simulink model "QaternionModel"  (R2012b)
settings: Solver=ode45  StartTime=0.0  StopTime=20  RelTol=1e-3
libraries: aerolibutil x6, aerolibtransform2 x6, vrlib x2, dspmtrx3 x1
settings Model: Creator=Mirag_000  LastModifiedBy=Mirag_000
settings DataIOCC: SignalLoggingSaveFormat=ModelDataLogs
settings OptimizationCC: ExpressionDepthLimit=128
settings DebuggingCC: MultiTaskDSMMsg=warning  MultiTaskCondExecSysMsg=none  StrictBusMsg=None
settings RTWCC: IncludeERTFirstTime=on
settings CodeAppCC: CustomSymbolStrType=$N$R$M_T  InternalIdentifier=Shortened

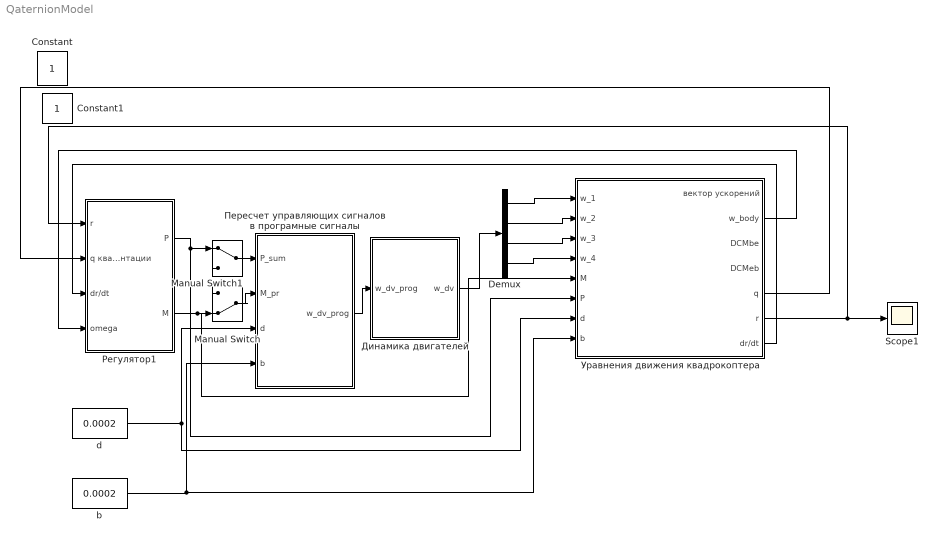
== system QaternionModel ==
  Demux : Demux
  Manual Switch : ManualSwitch  CurrentSetting=0
  Manual Switch1 : ManualSwitch
  Scope1 : Scope
  b : Constant  Value=0.0002
  d : Constant  Value=0.0002
  Динамика двигателей : Subsystem
  Пересчет управляющих сигналов в програмные сигналы : Subsystem
  Регулятор1 : Subsystem
  Уравнения движения квадрокоптера : Subsystem
  Constant : Constant  IOType=siggen  VectorParams1D=off  SampleTime=1
  Constant1 : Constant  IOType=siggen
  wires:
  Demux/1 -> Уравнения движения квадрокоптера/1(w_1)
  Demux/2 -> Уравнения движения квадрокоптера/2(w_2)
  Demux/3 -> Уравнения движения квадрокоптера/3(w_3)
  Demux/4 -> Уравнения движения квадрокоптера/4(w_4)
  Уравнения движения квадрокоптера/6(r) -> Регулятор1/1(r), Scope1/1
  Пересчет управляющих сигналов в програмные сигналы/1(w_dv_prog) -> Динамика двигателей/1(w_dv_prog)
  Уравнения движения квадрокоптера/5(q) -> Регулятор1/2(q кватернион текущей ориентации)
  Уравнения движения квадрокоптера/7(dr/dt) -> Регулятор1/3(dr/dt)
  Уравнения движения квадрокоптера/2(w_body) -> Регулятор1/4(omega)
  Регулятор1/1(P) -> Manual Switch1/1, Уравнения движения квадрокоптера/6(P)
  Регулятор1/2(M) -> Уравнения движения квадрокоптера/5(M), Manual Switch/2
  Динамика двигателей/1(w_dv) -> Demux/1
  Manual Switch1/1 -> Пересчет управляющих сигналов в програмные сигналы/1(P_sum)
  Manual Switch/1 -> Пересчет управляющих сигналов в програмные сигналы/2(M_pr)
  d/1 -> Пересчет управляющих сигналов в програмные сигналы/3(d), Уравнения движения квадрокоптера/7(d)
  b/1 -> Уравнения движения квадрокоптера/8(b), Пересчет управляющих сигналов в програмные сигналы/4(b)

== system QaternionModel/Динамика двигателей ==
  w_dv_prog : Inport
  Demux1 : Demux
  Manual Switch : ManualSwitch
  Scope : Scope
      settings: SaveName=ScopeData32
  Transfer Fcn{4..7} (4 alike) : TransferFcn  Denominator=[0.003 1]
  Vector Concatenate1 : Concatenate  NumInputs=4
  w_dv : Outport
  wires:
  Manual Switch/1 -> w_dv/1
  w_dv_prog/1 -> Demux1/1
  Transfer Fcn5/1 -> Vector Concatenate1/2
  Transfer Fcn6/1 -> Vector Concatenate1/3
  Transfer Fcn7/1 -> Vector Concatenate1/4
  Demux1/1 -> Transfer Fcn4/1
  Transfer Fcn4/1 -> Vector Concatenate1/1
  Demux1/2 -> Transfer Fcn5/1
  Demux1/3 -> Transfer Fcn6/1
  Demux1/4 -> Transfer Fcn7/1
  Vector Concatenate1/1 -> Scope/1, Manual Switch/1

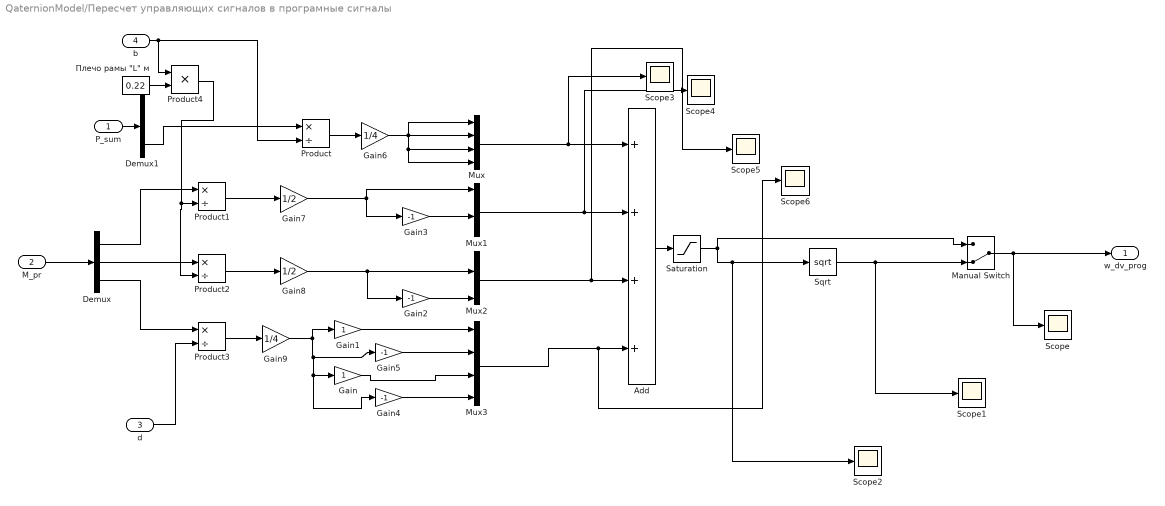
== system QaternionModel/Пересчет управляющих сигналов в програмные сигналы ==
  P_sum : Inport
  M_pr : Inport  Port=2
  d : Inport  Port=3
  b : Inport  Port=4
  Add : Sum  Inputs=++++
  Demux : Demux  Outputs=3
  Demux1 : Demux  Outputs=3
  Gain : Gain
  Gain1 : Gain
  Gain{2..5} (4 alike) : Gain  Gain=-1
  Gain6 : Gain  Gain=1/4
  Gain7 : Gain  Gain=1/2
  Gain8 : Gain  Gain=1/2
  Gain9 : Gain  Gain=1/4
  Manual Switch : ManualSwitch  CurrentSetting=0
  Mux{,1..3} (4 alike) : Mux
  Product{,1..3} (4 alike) : Product  Inputs=*/
  Product4 : Product
  Saturation : Saturate  UpperLimit=50000  LowerLimit=0.001
  Scope{,1..6} (7 alike) : Scope
      Scope settings: YMin=1.6575  YMax=1.6775  SaveName=ScopeData20
      Scope1 settings: YMin=60  YMax=180  SaveName=ScopeData34
      Scope2 settings: YMin=0.07  YMax=0.1025  SaveName=ScopeData44
      Scope3 settings: YMin=60  YMax=180  SaveName=ScopeData23
      Scope4 settings: YMin=60  YMax=180  SaveName=ScopeData24
      Scope5 settings: YMin=60  YMax=180  SaveName=ScopeData27
      Scope6 settings: YMin=60  YMax=180  SaveName=ScopeData28
  Sqrt : Sqrt  SaturateOnIntegerOverflow=on
  "Плечо рамы \"L\" м" : Constant  Value=0.22
  w_dv_prog : Outport
  wires:
  Gain/1 -> Mux3/3
  Gain1/1 -> Mux3/1
  Product3/1 -> Gain9/1
  Product2/1 -> Gain8/1
  Gain2/1 -> Mux2/4
  Gain3/1 -> Mux1/3
  Product1/1 -> Gain7/1
  Product/1 -> Gain6/1
  Mux2/1 -> Scope5/1, Add/3
  Mux1/1 -> Scope4/1, Add/2
  Mux/1 -> Scope3/1, Add/1
  Mux3/1 -> Scope6/1, Add/4
  Gain5/1 -> Mux3/2
  Gain4/1 -> Mux3/4
  Sqrt/1 -> Scope1/1, Manual Switch/2
  Demux/1 -> Product1/1
  Demux/2 -> Product2/1
  d/1 -> Product3/2
  "Плечо рамы \"L\" м"/1 -> Product4/2
  b/1 -> Product/2, Product4/1
  Product4/1 -> Product2/2, Product1/2
  Gain6/1 -> Mux/4, Mux/3, Mux/1, Mux/2
  Gain7/1 -> Gain3/1, Mux1/1
  Gain8/1 -> Gain2/1, Mux2/2
  Gain9/1 -> Gain1/1, Gain4/1, Gain/1, Gain5/1
  Demux/3 -> Product3/1
  M_pr/1 -> Demux/1
  P_sum/1 -> Demux1/1
  Demux1/3 -> Product/1
  Manual Switch/1 -> w_dv_prog/1, Scope/1
  Add/1 -> Saturation/1
  Saturation/1 -> Manual Switch/1, Scope2/1, Sqrt/1

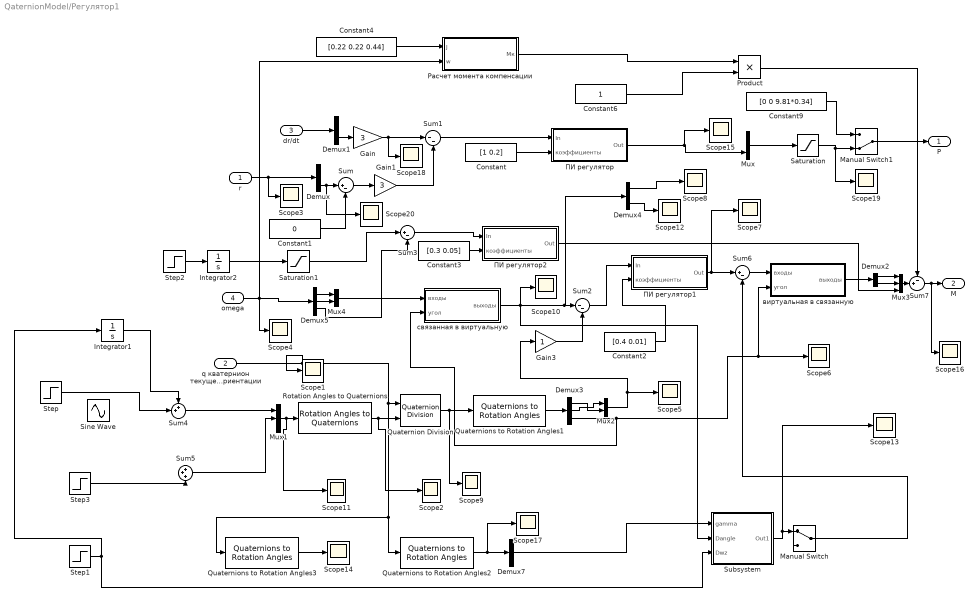
== system QaternionModel/Регулятор1 ==
  r : Inport
  q кватернион текущей ориентации : Inport  Port=2
  dr/dt : Inport  Port=3
  omega : Inport  Port=4
  Constant : Constant  Value=[1 0.2]
  Constant1 : Constant  Value=0
  Constant2 : Constant  Value=[0.4 0.01]
  Constant3 : Constant  Value=[0.3 0.05]
  Constant4 : Constant  Value=[0.22 0.22 0.44]
  Constant6 : Constant
  Constant9 : Constant  Value=[0 0 9.81*0.34]
  Demux{,1,3,5,7} (5 alike) : Demux  Outputs=3
  Demux2 : Demux  Outputs=2
  Demux4 : Demux  Outputs=2
  Gain : Gain  Gain=3
  Gain1 : Gain  Gain=3
  Gain3 : Gain
  Integrator1 : Integrator
  Integrator2 : Integrator
  Manual Switch : ManualSwitch
  Manual Switch1 : ManualSwitch  CurrentSetting=0
  Mux : Mux  Inputs=3
  Mux1 : Mux  Inputs=3
  Mux2 : Mux  Inputs=2
  Mux3 : Mux  Inputs=3
  Mux4 : Mux  Inputs=2
  Product : Product  RndMeth=Zero
  Quaternion Division : aerolibutil/Quaternion Division
  Quaternions to Rotation Angles1 : aerolibtransform2/Quaternions to Rotation Angles  rotationOrder=YXZ
  Quaternions to Rotation Angles2 : aerolibtransform2/Quaternions to Rotation Angles  rotationOrder=ZYZ
  Quaternions to Rotation Angles3 : aerolibtransform2/Quaternions to Rotation Angles  rotationOrder=ZYZ
  Rotation Angles to Quaternions : aerolibtransform2/Rotation Angles to Quaternions  rotationOrder=ZYX
  Saturation : Saturate  UpperLimit=100  LowerLimit=0
  Saturation1 : Saturate  UpperLimit=3  LowerLimit=0
  Scope{1..20} (20 alike) : Scope
      Scope1 settings: SaveName=ScopeData2
      Scope10 settings: YMin=-0.008  YMax=0.008  SaveName=ScopeData12
      Scope11 settings: YMin=-1  YMax=0.1  SaveName=ScopeData14
      Scope12 settings: YMin=-2.75  YMax=1.5  SaveName=ScopeData17
      Scope13 settings: YMin=-2.75  YMax=1.5  SaveName=ScopeData21
      Scope14 settings: TimeRange=18.29822608393934  YMin=0.993671875  YMax=1.008984375  SaveName=ScopeData22
      Scope15 settings: YMin=-2.75  YMax=1.5  SaveName=ScopeData10
      Scope16 settings: YMin=-2.75  YMax=1.5  SaveName=ScopeData29
      Scope17 settings: TimeRange=18.29822608393934  YMin=0.993671875  YMax=1.008984375  SaveName=ScopeData25
      Scope18 settings: SaveName=ScopeData30
      Scope19 settings: TimeRange=20  YMin=-2.75  YMax=1.5  SaveName=ScopeData31
      Scope2 settings: YMin=-1  YMax=0.1  SaveName=ScopeData3
      Scope20 settings: SaveName=ScopeData33
      Scope3 settings: SaveName=ScopeData5
      Scope4 settings: YMin=-0.01  YMax=0.11  SaveName=ScopeData4
      Scope5 settings: TimeRange=400  YMin=1.38778e-17  YMax=0.275  SaveName=ScopeData7
      Scope6 settings: YMin=-2.75  YMax=1.5  SaveName=ScopeData8
      Scope7 settings: YMin=-2.75  YMax=1.5  SaveName=ScopeData9
      Scope8 settings: YMin=-2.75  YMax=1.5  SaveName=ScopeData16
      Scope9 settings: YMin=-1  YMax=0.1  SaveName=ScopeData11
  Sine Wave : Sin  Amplitude=0  Frequency=0.2  SampleTime=0
  Step : Step  Time=3  After=0.1  SampleTime=4
  Step1 : Step  Time=2  After=0.5  SampleTime=0
  Step2 : Step  After=0.3  SampleTime=0
  Step3 : Step  After=0.5  SampleTime=0
  Subsystem : Subsystem
  Sum : Sum  Inputs=|+-
  Sum1 : Sum  Inputs=|--
  Sum2 : Sum  Inputs=|--
  Sum3 : Sum  Inputs=|+-
  Sum4 : Sum  Inputs=++|
  Sum5 : Sum  Inputs=+++
  Sum6 : Sum  Inputs=|+-
  Sum7 : Sum  Inputs=-+|
  ПИ регулятор : Subsystem
  ПИ регулятор1 : Subsystem
  ПИ регулятор2 : Subsystem
  Расчет момента компенсации : Subsystem
  виртуальная в связанную : Subsystem
  связанная в виртуальную : Subsystem
  P : Outport
  M : Outport  Port=2
  wires:
  r/1 -> Scope3/1, Demux/1
  dr/dt/1 -> Demux1/1
  Constant/1 -> ПИ регулятор/2(коэффициенты)
  Demux/3 -> Scope20/1, Sum/1
  Sum/1 -> Gain1/1
  Constant1/1 -> Sum/2
  Gain1/1 -> Sum1/2
  Sum1/1 -> ПИ регулятор/1(In)
  Mux/1 -> Saturation/1
  ПИ регулятор/1(Out) -> Scope15/1, Mux/3
  q кватернион текущей ориентации/1 -> Scope1/1, Quaternions to Rotation Angles3/1, Quaternions to Rotation Angles2/1, Quaternion Division/1
  Rotation Angles to Quaternions/1 -> Scope2/1, Quaternion Division/2
  Quaternions to Rotation Angles1/1 -> Demux3/1
  Quaternion Division/1 -> Scope9/1, Quaternions to Rotation Angles1/1
  Mux1/1 -> Scope11/1, Rotation Angles to Quaternions/1
  Mux2/1 -> Gain3/1, Scope5/1
  виртуальная в связанную/1(выходы) -> Demux2/1
  Demux3/3 -> связанная в виртуальную/2(угол), Scope6/1, виртуальная в связанную/2(угол)
  связанная в виртуальную/1(выходы) -> Subsystem/2(Dangle), Scope10/1, Demux4/1, Sum2/1
  Gain3/1 -> Sum2/2
  Constant2/1 -> ПИ регулятор1/2(коэффициенты)
  ПИ регулятор1/1(Out) -> Sum6/1, Scope7/1
  Demux5/1 -> Mux4/1
  Demux5/2 -> Mux4/2
  Mux4/1 -> связанная в виртуальную/1(входы)
  omega/1 -> Расчет момента компенсации/2(w), Scope4/1, Demux5/1
  Constant3/1 -> ПИ регулятор2/2(коэффициенты)
  Sum3/1 -> ПИ регулятор2/1(In)
  Demux5/3 -> Sum3/2
  ПИ регулятор2/1(Out) -> Mux3/3
  Sum5/1 -> Mux1/2
  Demux4/1 -> Scope8/1
  Demux4/2 -> Scope12/1
  Step3/1 -> Sum5/3
  Demux2/1 -> Mux3/1
  Demux2/2 -> Mux3/2
  Quaternions to Rotation Angles2/1 -> Scope17/1, Demux7/1
  Demux3/1 -> Mux2/2
  Demux3/2 -> Mux2/1
  Sum2/1 -> ПИ регулятор1/1(In)
  Sum4/1 -> Mux1/1
  Demux7/2 -> Subsystem/1(gamma)
  Integrator1/1 -> Sum4/1
  Step1/1 -> Subsystem/3(Dwz), Integrator1/1
  Subsystem/1(Out1) -> Scope13/1, Manual Switch/1
  Quaternions to Rotation Angles3/1 -> Scope14/1
  Sum6/1 -> виртуальная в связанную/1(входы)
  Manual Switch/1 -> Sum6/2
  Step/1 -> Sum4/2
  Mux3/1 -> Sum7/2
  Sum7/1 -> Scope16/1, M/1
  Constant4/1 -> Расчет момента компенсации/1(J)
  Product/1 -> Sum7/1
  Расчет момента компенсации/1(Мк) -> Product/1
  Constant6/1 -> Product/2
  Saturation/1 -> Manual Switch1/2, Scope19/1
  Demux1/3 -> Gain/1
  Gain/1 -> Scope18/1, Sum1/1
  Manual Switch1/1 -> P/1
  Constant9/1 -> Manual Switch1/1
  Step2/1 -> Integrator2/1
  Integrator2/1 -> Saturation1/1
  Saturation1/1 -> Sum3/1

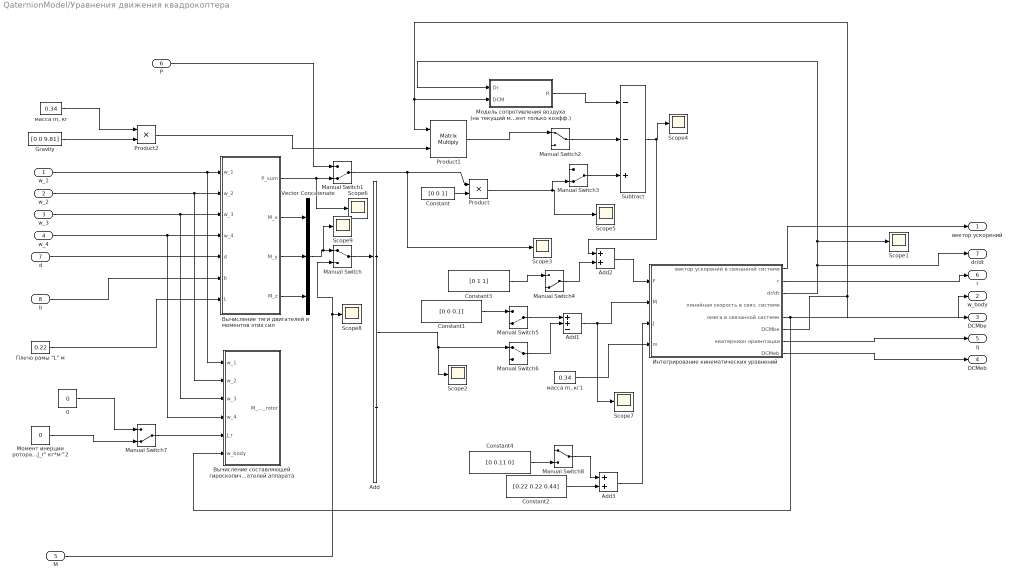
== system QaternionModel/Уравнения движения квадрокоптера ==
  w_1 : Inport
  w_2 : Inport  Port=2
  w_3 : Inport  Port=3
  w_4 : Inport  Port=4
  M : Inport  Port=5
  P : Inport  Port=6
  d : Inport  Port=7
  b : Inport  Port=8
  0 : Constant  Value=0
  Add : Sum  Inputs=+-
  Add1 : Sum  Inputs=++-
  Add2 : Sum
  Add3 : Sum
  Constant : Constant  Value=[0 0 1]
  Constant1 : Constant  Value=[0 0 0.1]
  Constant2 : Constant  Value=[0.22 0.22 0.44]
  Constant3 : Constant  Value=[0 1 1]
  Constant4 : Constant  Value=[0 0.11 0]
  Gravity : Constant  Value=[0 0 9.81]
  Manual Switch{,2,6,8} (4 alike) : ManualSwitch
  Manual Switch{1,3..5,7} (5 alike) : ManualSwitch  CurrentSetting=0
  Product : Product
  Product1 : Product  Multiplication=Matrix(*)  RndMeth=Zero
  Product2 : Product  RndMeth=Zero
  Scope{1..9} (9 alike) : Scope
      Scope2 settings: SaveName=ScopeData13
      Scope3 settings: YMin=0  YMax=60  SaveName=ScopeData41
      Scope4 settings: SaveName=ScopeData18
      Scope5 settings: TimeRange=20  YMin=-1  YMax=1  SaveName=ScopeData19
      Scope6 settings: TimeRange=20  YMin=-1  YMax=1  SaveName=ScopeData37
      Scope7 settings: SaveName=ScopeData15
      Scope8 settings: SaveName=ScopeData38
      Scope9 settings: SaveName=ScopeData39
  Subtract : Sum  Inputs=--+
  Vector Concatenate : Concatenate  NumInputs=3
  Вычисление составляющей гироскопического момента роторов двигателей аппарата : Subsystem
  Вычисление тяги двигателей и моментов этих сил : Subsystem
  Интегрирование кинематических уравнений : Subsystem
  Модель сопротивления воздуха (на текущий момент только коэфф.) : Subsystem
  "Момент инерции ротора \"J_r\" кг*м^2" : Constant  Value=0
  "Плечо рамы \"L\" м" : Constant  Value=0.22
  "масса m, кг" : Constant  Value=0.34
  "масса m, кг1" : Constant  Value=0.34
  вектор ускорений : Outport
  w_body : Outport  Port=2
  "DCMbe " : Outport  Port=3
  DCMeb : Outport  Port=4
  q : Outport  Port=5
  r : Outport  Port=6
  dr/dt : Outport  Port=7
  wires:
  w_1/1 -> Вычисление составляющей гироскопического момента роторов двигателей аппарата/1(w_1), Вычисление тяги двигателей и моментов этих сил/1(w_1)
  w_2/1 -> Вычисление составляющей гироскопического момента роторов двигателей аппарата/2(w_2), Вычисление тяги двигателей и моментов этих сил/2(w_2)
  w_3/1 -> Вычисление тяги двигателей и моментов этих сил/3(w_3), Вычисление составляющей гироскопического момента роторов двигателей аппарата/3(w_3)
  w_4/1 -> Вычисление составляющей гироскопического момента роторов двигателей аппарата/4(w_4), Вычисление тяги двигателей и моментов этих сил/4(w_4)
  d/1 -> Вычисление тяги двигателей и моментов этих сил/5(d)
  b/1 -> Вычисление тяги двигателей и моментов этих сил/6(b)
  "Плечо рамы \"L\" м"/1 -> Вычисление тяги двигателей и моментов этих сил/7(L)
  Вычисление тяги двигателей и моментов этих сил/4(M_z) -> Vector Concatenate/3
  Constant/1 -> Product/2
  "масса m, кг"/1 -> Product2/1
  Модель сопротивления воздуха (на текущий момент только коэфф.)/1(R) -> Subtract/1
  Gravity/1 -> Product2/2
  Product2/1 -> Product1/2
  Subtract/1 -> Add2/1, Scope4/1
  Product/1 -> Manual Switch3/2, Scope5/1
  Интегрирование кинематических уравнений/5(омега в связанной системе) -> Вычисление составляющей гироскопического момента роторов двигателей аппарата/6(w_body), w_body/1
  Manual Switch/1 -> Add/1
  Vector Concatenate/1 -> Scope9/1, Manual Switch/1
  Вычисление тяги двигателей и моментов этих сил/1(P_sum) -> Scope6/1, Manual Switch1/2
  Manual Switch1/1 -> Scope3/1, Product/1
  Интегрирование кинематических уравнений/8(DCMeb) -> DCMeb/1
  Интегрирование кинематических уравнений/7("кватернион ориентации ") -> q/1
  Интегрирование кинематических уравнений/6(DCMbe) -> Product1/1, Модель сопротивления воздуха (на текущий момент только коэфф.)/2(DCM), "DCMbe "/1
  "масса m, кг1"/1 -> Интегрирование кинематических уравнений/4(m)
  Интегрирование кинематических уравнений/2(r) -> r/1
  Интегрирование кинематических уравнений/1(вектор ускорений в связанной системе) -> вектор ускорений/1
  Интегрирование кинематических уравнений/3(dr/dt) -> Модель сопротивления воздуха (на текущий момент только коэфф.)/1(Dr), Scope1/1, dr/dt/1
  Add2/1 -> Интегрирование кинематических уравнений/1(F)
  Manual Switch2/1 -> Subtract/2
  Product1/1 -> Manual Switch2/1
  Manual Switch3/1 -> Subtract/3
  Manual Switch4/1 -> Add2/2
  Constant3/1 -> Manual Switch4/1
  Add1/1 -> Scope7/1, Интегрирование кинематических уравнений/2(M)
  Manual Switch5/1 -> Add1/1
  Constant1/1 -> Manual Switch5/1
  Manual Switch6/1 -> Add1/2
  Add/1 -> Scope2/1, Manual Switch6/1
  Manual Switch7/1 -> Вычисление составляющей гироскопического момента роторов двигателей аппарата/5(J_r)
  "Момент инерции ротора \"J_r\" кг*м^2"/1 -> Manual Switch7/2
  0/1 -> Manual Switch7/1
  Constant2/1 -> Add3/2
  Add3/1 -> Интегрирование кинематических уравнений/3(J)
  Constant4/1 -> Manual Switch8/2
  Manual Switch8/1 -> Add3/1
  P/1 -> Manual Switch1/1
  M/1 -> Manual Switch/2, Scope8/1
  Вычисление тяги двигателей и моментов этих сил/2(M_x) -> Vector Concatenate/1
  Вычисление тяги двигателей и моментов этих сил/3(M_y) -> Vector Concatenate/2

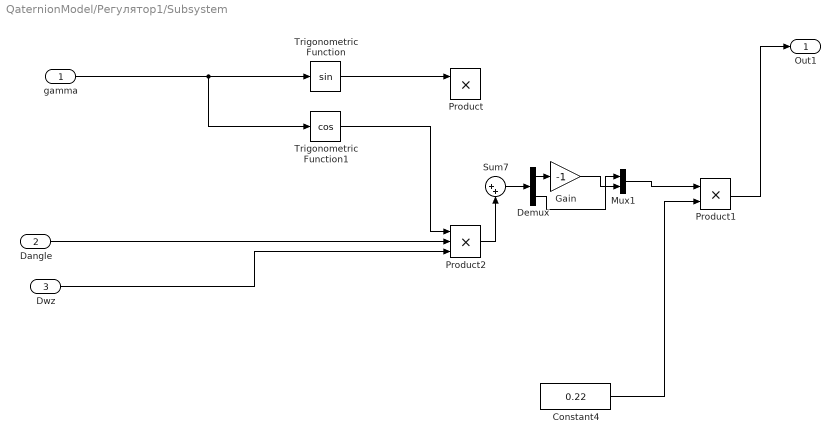
== system QaternionModel/Регулятор1/Subsystem ==
  gamma : Inport
  Dangle : Inport  Port=2
  Dwz : Inport  Port=3
  Constant4 : Constant  Value=0.22
  Demux : Demux  Outputs=2
  Gain : Gain  Gain=-1
  Mux1 : Mux  Inputs=2
  Product : Product  RndMeth=Zero
  Product1 : Product  RndMeth=Zero
  Product2 : Product  Inputs=3  RndMeth=Zero
  Sum7 : Sum  Inputs=|++
  Trigonometric Function : Trigonometry
  Trigonometric Function1 : Trigonometry  Operator=cos
  Out1 : Outport
  wires:
  Product1/1 -> Out1/1
  Constant4/1 -> Product1/2
  Trigonometric Function/1 -> Product/1
  gamma/1 -> Trigonometric Function1/1, Trigonometric Function/1
  Product2/1 -> Sum7/2
  Trigonometric Function1/1 -> Product2/1
  Dwz/1 -> Product2/3
  Dangle/1 -> Product2/2
  Sum7/1 -> Demux/1
  Demux/1 -> Gain/1
  Gain/1 -> Mux1/2
  Demux/2 -> Mux1/1
  Mux1/1 -> Product1/1

== system QaternionModel/Регулятор1/ПИ регулятор ==
  In : Inport
  коэффициенты : Inport  Port=2
  Add : Sum
  Demux : Demux  Outputs=2
  Integrator : Integrator
  Product : Product  RndMeth=Zero
  Product1 : Product  RndMeth=Zero
  Out : Outport
  wires:
  коэффициенты/1 -> Demux/1
  Add/1 -> Out/1
  Product/1 -> Add/1
  In/1 -> Integrator/1, Product/1
  Demux/1 -> Product/2
  Product1/1 -> Add/2
  Demux/2 -> Product1/2
  Integrator/1 -> Product1/1

== system QaternionModel/Регулятор1/ПИ регулятор1 ==
  In : Inport
  коэффициенты : Inport  Port=2
  Add : Sum  Inputs=+++
  Demux : Demux  Outputs=2
  Integrator : Integrator
  Product : Product  RndMeth=Zero
  Product1 : Product  RndMeth=Zero
  Out : Outport
  wires:
  коэффициенты/1 -> Demux/1
  Add/1 -> Out/1
  Product/1 -> Add/1
  In/1 -> Integrator/1, Product/1
  Demux/1 -> Product/2
  Demux/2 -> Product1/2
  Integrator/1 -> Product1/1
  Product1/1 -> Add/2

== system QaternionModel/Регулятор1/ПИ регулятор2 ==
  In : Inport
  коэффициенты : Inport  Port=2
  Add : Sum
  Demux : Demux  Outputs=2
  Integrator : Integrator
  Product : Product  RndMeth=Zero
  Product1 : Product  RndMeth=Zero
  Out : Outport
  wires:
  коэффициенты/1 -> Demux/1
  Add/1 -> Out/1
  Product/1 -> Add/1
  In/1 -> Integrator/1, Product/1
  Demux/1 -> Product/2
  Product1/1 -> Add/2
  Demux/2 -> Product1/2
  Integrator/1 -> Product1/1

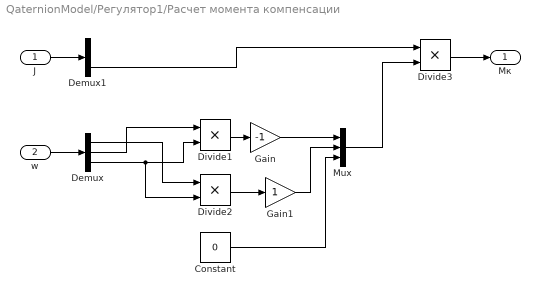
== system QaternionModel/Регулятор1/Расчет момента компенсации ==
  J : Inport
  w : Inport  Port=2
  Constant : Constant  Value=0
  Demux : Demux  Outputs=3
  Demux1 : Demux  Outputs=3
  Divide1 : Product  Inputs=**
  Divide2 : Product  Inputs=**
  Divide3 : Product  Inputs=**
  Gain : Gain  Gain=-1
  Gain1 : Gain
  Mux : Mux  Inputs=3
  Мк : Outport
  wires:
  w/1 -> Demux/1
  J/1 -> Demux1/1
  Demux/3 -> Divide2/2, Divide1/2
  Demux/1 -> Divide2/1
  Demux/2 -> Divide1/1
  Divide1/1 -> Gain/1
  Divide2/1 -> Gain1/1
  Gain/1 -> Mux/1
  Constant/1 -> Mux/3
  Mux/1 -> Divide3/2
  Demux1/3 -> Divide3/1
  Divide3/1 -> Мк/1
  Gain1/1 -> Mux/2

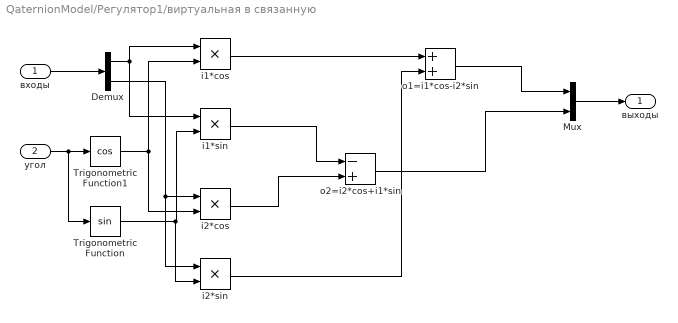
== system QaternionModel/Регулятор1/виртуальная в связанную ==
  входы : Inport
  угол : Inport  Port=2
  Demux : Demux  Outputs=2
  Mux : Mux  Inputs=2
  Trigonometric Function : Trigonometry
  Trigonometric Function1 : Trigonometry  Operator=cos
  i1*cos : Product  RndMeth=Zero
  i1*sin : Product  RndMeth=Zero
  i2*cos : Product  RndMeth=Zero
  i2*sin : Product  RndMeth=Zero
  o1=i1*cos-i2*sin : Sum
  o2=i2*cos+i1*sin : Sum  Inputs=-+
  выходы : Outport
  wires:
  угол/1 -> Trigonometric Function/1, Trigonometric Function1/1
  входы/1 -> Demux/1
  Trigonometric Function/1 -> i2*sin/2, i1*sin/2
  Trigonometric Function1/1 -> i1*cos/2, i2*cos/2
  Demux/1 -> i1*sin/1, i1*cos/1
  Demux/2 -> i2*sin/1, i2*cos/1
  Mux/1 -> выходы/1
  i2*cos/1 -> o2=i2*cos+i1*sin/2
  i1*sin/1 -> o2=i2*cos+i1*sin/1
  i1*cos/1 -> o1=i1*cos-i2*sin/1
  i2*sin/1 -> o1=i1*cos-i2*sin/2
  o2=i2*cos+i1*sin/1 -> Mux/2
  o1=i1*cos-i2*sin/1 -> Mux/1

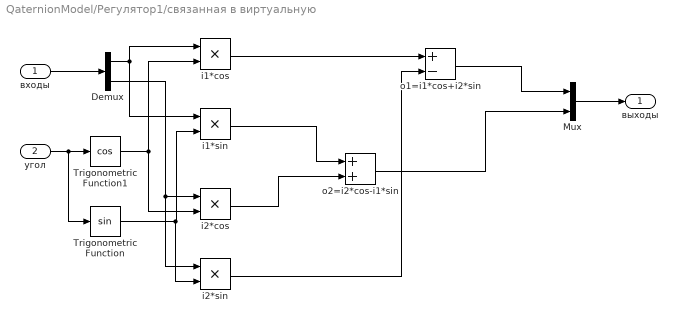
== system QaternionModel/Регулятор1/связанная в виртуальную ==
  входы : Inport
  угол : Inport  Port=2
  Demux : Demux  Outputs=2
  Mux : Mux  Inputs=2
  Trigonometric Function : Trigonometry
  Trigonometric Function1 : Trigonometry  Operator=cos
  i1*cos : Product  RndMeth=Zero
  i1*sin : Product  RndMeth=Zero
  i2*cos : Product  RndMeth=Zero
  i2*sin : Product  RndMeth=Zero
  o1=i1*cos+i2*sin : Sum  Inputs=+-
  o2=i2*cos-i1*sin : Sum
  выходы : Outport
  wires:
  угол/1 -> Trigonometric Function/1, Trigonometric Function1/1
  входы/1 -> Demux/1
  Trigonometric Function/1 -> i2*sin/2, i1*sin/2
  Trigonometric Function1/1 -> i1*cos/2, i2*cos/2
  Demux/1 -> i1*sin/1, i1*cos/1
  Demux/2 -> i2*sin/1, i2*cos/1
  Mux/1 -> выходы/1
  i2*cos/1 -> o2=i2*cos-i1*sin/2
  i1*sin/1 -> o2=i2*cos-i1*sin/1
  i1*cos/1 -> o1=i1*cos+i2*sin/1
  i2*sin/1 -> o1=i1*cos+i2*sin/2
  o2=i2*cos-i1*sin/1 -> Mux/2
  o1=i1*cos+i2*sin/1 -> Mux/1

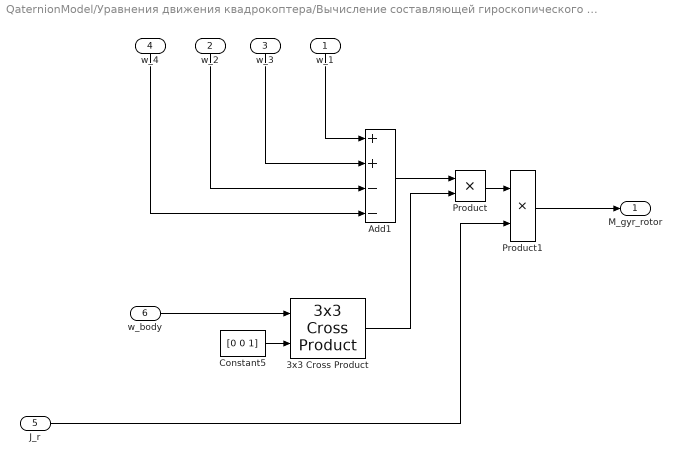
== system QaternionModel/Уравнения движения квадрокоптера/Вычисление составляющей гироскопического момента роторов двигателей аппарата ==
  w_1 : Inport
  w_2 : Inport  Port=2
  w_3 : Inport  Port=3
  w_4 : Inport  Port=4
  J_r : Inport  Port=5
  w_body : Inport  Port=6
  3x3 Cross Product : aerolibutil/3x3 Cross Product
  Add1 : Sum  Inputs=++--
  Constant5 : Constant  Value=[0 0 1]
  Product : Product
  Product1 : Product
  M_gyr_rotor : Outport
  wires:
  Add1/1 -> Product/1
  3x3 Cross Product/1 -> Product/2
  w_body/1 -> 3x3 Cross Product/1
  Constant5/1 -> 3x3 Cross Product/2
  J_r/1 -> Product1/2
  Product/1 -> Product1/1
  Product1/1 -> M_gyr_rotor/1
  w_2/1 -> Add1/3
  w_3/1 -> Add1/2
  w_1/1 -> Add1/1
  w_4/1 -> Add1/4

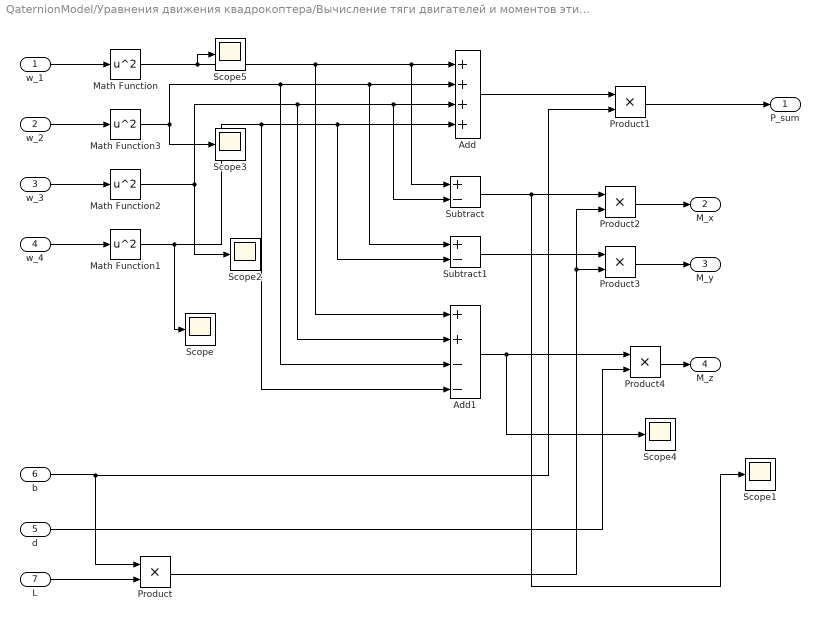
== system QaternionModel/Уравнения движения квадрокоптера/Вычисление тяги двигателей и моментов этих сил ==
  w_1 : Inport
  w_2 : Inport  Port=2
  w_3 : Inport  Port=3
  w_4 : Inport  Port=4
  d : Inport  Port=5
  b : Inport  Port=6
  L : Inport  Port=7
  Add : Sum  Inputs=++++
  Add1 : Sum  Inputs=++--
  Math Function{,1..3} (4 alike) : Math  Operator=square  SaturateOnIntegerOverflow=on
  Product{,1..4} (5 alike) : Product
  Scope{,1..5} (6 alike) : Scope
      Scope settings: YMin=2.5  YMax=42.5  SaveName=ScopeData43
      Scope1 settings: YMin=0.135  YMax=0.205  SaveName=ScopeData45
      Scope2 settings: YMin=2.5  YMax=42.5  SaveName=ScopeData35
      Scope3 settings: YMin=2.5  YMax=42.5  SaveName=ScopeData36
      Scope4 settings: YMin=0.135  YMax=0.205  SaveName=ScopeData40
      Scope5 settings: YMin=2.5  YMax=42.5  SaveName=ScopeData42
  Subtract : Sum  Inputs=+-
  Subtract1 : Sum  Inputs=+-
  P_sum : Outport
  M_x : Outport  Port=2
  M_y : Outport  Port=3
  M_z : Outport  Port=4
  wires:
  w_1/1 -> Math Function/1
  w_4/1 -> Math Function1/1
  w_3/1 -> Math Function2/1
  w_2/1 -> Math Function3/1
  Math Function/1 -> Scope5/1, Add1/1, Subtract/1, Add/1
  Math Function3/1 -> Subtract1/1, Add/2, Add1/3, Scope3/1
  Math Function2/1 -> Subtract/2, Add/3, Add1/2, Scope2/1
  Math Function1/1 -> Scope/1, Subtract1/2, Add/4, Add1/4
  b/1 -> Product1/2, Product/1
  L/1 -> Product/2
  Add/1 -> Product1/1
  Product2/1 -> M_x/1
  Subtract/1 -> Scope1/1, Product2/1
  Subtract1/1 -> Product3/1
  Product/1 -> Product2/2, Product3/2
  Product3/1 -> M_y/1
  Add1/1 -> Scope4/1, Product4/1
  d/1 -> Product4/2
  Product4/1 -> M_z/1
  Product1/1 -> P_sum/1

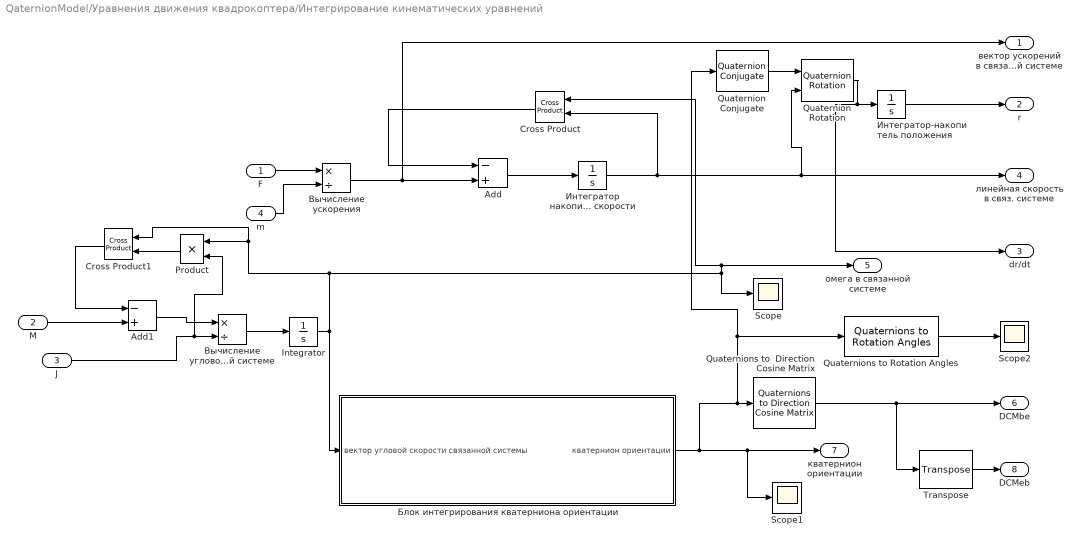
== system QaternionModel/Уравнения движения квадрокоптера/Интегрирование кинематических уравнений ==
  F : Inport
  M : Inport  Port=2
  J : Inport  Port=3
  m : Inport  Port=4
  Add : Sum  Inputs=-+
  Add1 : Sum  Inputs=-+
  Cross Product : vrlib/Utilities/Cross Product
  Cross Product1 : vrlib/Utilities/Cross Product
  Integrator : Integrator  InitialCondition=[0 0 0]
  Product : Product  RndMeth=Zero
  Quaternion Conjugate : aerolibutil/Quaternion Conjugate
  Quaternion Rotation : aerolibutil/Quaternion Rotation
  Quaternions to  Direction Cosine Matrix : aerolibtransform2/Quaternions to  Direction Cosine Matrix
  Quaternions to Rotation Angles : aerolibtransform2/Quaternions to Rotation Angles  rotationOrder=ZXZ
  Scope : Scope
      settings: SaveName=ScopeData6
  Scope1 : Scope
      settings: YMin=-0.01  YMax=0.01  SaveName=ScopeData26
  Scope2 : Scope
      settings: YMin=-3.5  YMax=3.5  SaveName=ScopeData73
  Transpose : dspmtrx3/Transpose  Hermitian=off  overflowFlag=off
  Блок интегрирования кватерниона ориентации : Subsystem
  Вычисление углового ускорения в связанной системе : Product  Inputs=*/
  Вычисление ускорения : Product  Inputs=*/
  Интегратор накопитель линейной скорости : Integrator  InitialCondition=[0 0 0]
  Интегратор-накопитель положения : Integrator
  вектор ускорений в связанной системе : Outport
  r : Outport  Port=2
  dr/dt : Outport  Port=3
  линейная скорость в связ. системе : Outport  Port=4
  омега в связанной системе : Outport  Port=5
  DCMbe : Outport  Port=6
  "кватернион ориентации " : Outport  Port=7
  DCMeb : Outport  Port=8
  wires:
  J/1 -> Product/2, Вычисление углового ускорения в связанной системе/2
  Вычисление углового ускорения в связанной системе/1 -> Integrator/1
  Integrator/1 -> Scope/1, омега в связанной системе/1, Cross Product/1, Cross Product1/1, Product/1, Блок интегрирования кватерниона ориентации/1(вектор угловой скорости связанной системы)
  Блок интегрирования кватерниона ориентации/1(кватернион ориентации) -> Quaternion Conjugate/1, Quaternions to Rotation Angles/1, Quaternions to  Direction Cosine Matrix/1, Scope1/1, "кватернион ориентации "/1
  Quaternions to  Direction Cosine Matrix/1 -> Transpose/1, DCMbe/1
  Transpose/1 -> DCMeb/1
  Quaternions to Rotation Angles/1 -> Scope2/1
  m/1 -> Вычисление ускорения/2
  F/1 -> Вычисление ускорения/1
  Вычисление ускорения/1 -> вектор ускорений в связанной системе/1, Add/2
  Add/1 -> Интегратор накопитель линейной скорости/1
  Интегратор накопитель линейной скорости/1 -> Cross Product/2, Quaternion Rotation/2, линейная скорость в связ. системе/1
  Cross Product/1 -> Add/1
  Интегратор-накопитель положения/1 -> r/1
  Quaternion Rotation/1 -> dr/dt/1, Интегратор-накопитель положения/1
  Quaternion Conjugate/1 -> Quaternion Rotation/1
  M/1 -> Add1/2
  Cross Product1/1 -> Add1/1
  Add1/1 -> Вычисление углового ускорения в связанной системе/1
  Product/1 -> Cross Product1/2

== system QaternionModel/Уравнения движения квадрокоптера/Модель сопротивления воздуха (на текущий момент только коэфф.) ==
  Dr : Inport
  DCM : Inport  Port=2
  Gain : Gain  Gain=0
  Product : Product  Multiplication=Matrix(*)  RndMeth=Zero
  R : Outport
  wires:
  Dr/1 -> Gain/1
  Product/1 -> R/1
  Gain/1 -> Product/2
  DCM/1 -> Product/1

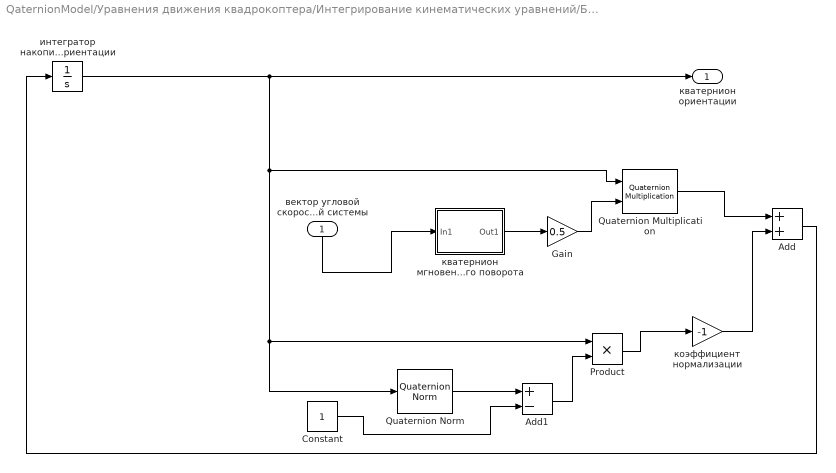
== system QaternionModel/Уравнения движения квадрокоптера/Интегрирование кинематических уравнений/Блок интегрирования кватерниона ориентации ==
  вектор угловой скорости связанной системы : Inport
  Add : Sum
  Add1 : Sum  Inputs=+-
  Constant : Constant
  Gain : Gain  Gain=0.5
  Product : Product  RndMeth=Zero
  Quaternion Multiplication : aerolibutil/Quaternion Multiplication
  Quaternion Norm : aerolibutil/Quaternion Norm
  интегратор накопитель кватерниона ориентации : Integrator  InitialCondition=[1 0 0 0]
  кватернион мгновенного поворота : Subsystem
  коэффициент нормализации : Gain  Gain=-1
  кватернион ориентации : Outport
  wires:
  вектор угловой скорости связанной системы/1 -> кватернион мгновенного поворота/1(In1)
  Product/1 -> коэффициент нормализации/1
  интегратор накопитель кватерниона ориентации/1 -> кватернион ориентации/1, Quaternion Norm/1, Product/1, Quaternion Multiplication/1
  Gain/1 -> Quaternion Multiplication/2
  коэффициент нормализации/1 -> Add/2
  Quaternion Multiplication/1 -> Add/1
  Add/1 -> интегратор накопитель кватерниона ориентации/1
  кватернион мгновенного поворота/1(Out1) -> Gain/1
  Quaternion Norm/1 -> Add1/1
  Constant/1 -> Add1/2
  Add1/1 -> Product/2

== system QaternionModel/Уравнения движения квадрокоптера/Интегрирование кинематических уравнений/Блок интегрирования кватерниона ориентации/кватернион мгновенного поворота ==
  In1 : Inport
  Constant : Constant  Value=0
  Demux : Demux  Outputs=3
  Mux : Mux
  Out1 : Outport
  wires:
  In1/1 -> Demux/1
  Demux/3 -> Mux/4
  Demux/2 -> Mux/3
  Demux/1 -> Mux/2
  Constant/1 -> Mux/1
  Mux/1 -> Out1/1
